simulink model "model_try"  (R2025b)
settings: Solver=VariableStepAuto  StartTime=0.0  StopTime=5.0  RelTol=1e-3
undefined symbols (not defined in the file or in its folder): g, pow, R0
settings Model: SimulationMode=rapid-accelerator  Creator=velo  LastModifiedBy=velo

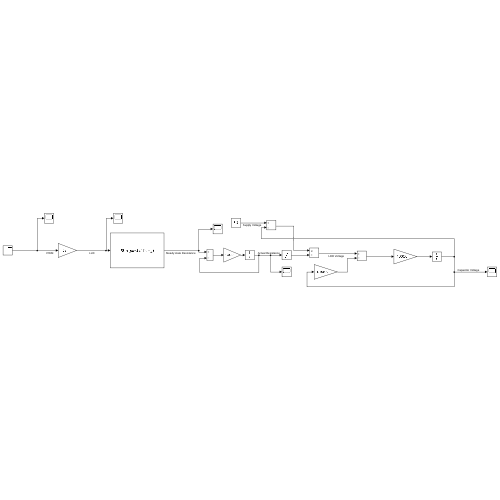
[thumbnail: Simulink's stored preview of the top-level diagram]
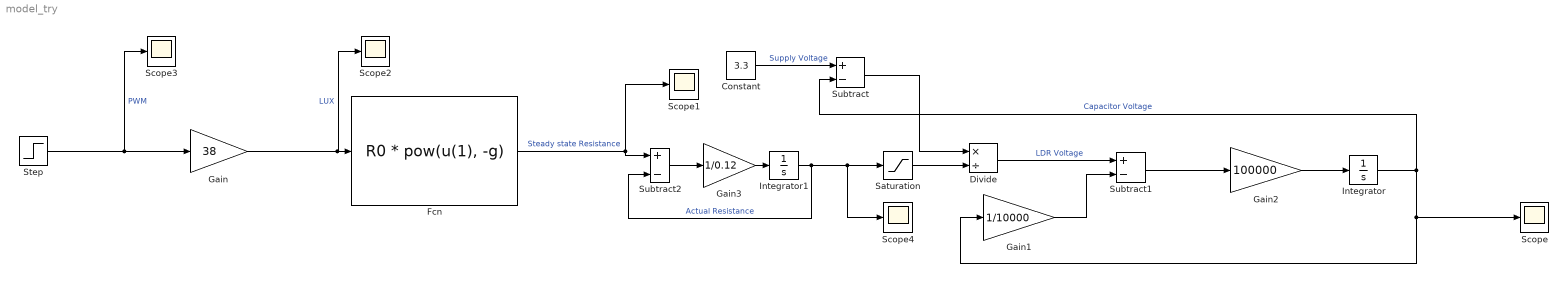
== system model_try ==
  Constant : Constant  Value=3.3
  Divide : Product  Inputs=*/
  Fcn : Fcn  Expr=R0 * pow(u(1), -g)
  Gain : Gain  Gain=38
  Gain1 : Gain  Gain=1/10000
  Gain2 : Gain  Gain=100000
  Gain3 : Gain  Gain=1/0.12
  Integrator : Integrator  InitialCondition=0.255
  Integrator1 : Integrator  InitialCondition=120000
  Saturation : Saturate  UpperLimit=inf  LowerLimit=100
  Scope{,1..4} (5 alike) : Scope
      Scope settings: ActiveDisplayYMinimum=0.22586838074123314  ActiveDisplayYMaximum=0.44234428417345445
      Scope1 settings: ActiveDisplayYMinimum=62371.168073078486  ActiveDisplayYMaximum=126049.34258955714
      Scope2 settings: ActiveDisplayYMinimum=16.625  ActiveDisplayYMaximum=40.375  DataLoggingVariableName=ScopeData2
      Scope3 settings: ActiveDisplayYMinimum=-1  ActiveDisplayYMaximum=1  DataLoggingVariableName=ScopeData3
      Scope4 settings: ActiveDisplayYMinimum=62331.451558114684  ActiveDisplayYMaximum=126407.61649354281  DataLoggingVariableName=ScopeData4
  Step : Step  Before=0.5  SampleTime=1
  Subtract : Sum  Inputs=+-
  Subtract1 : Sum  Inputs=+-
  Subtract2 : Sum  Inputs=+-
  wires:
  Step/1 -> Gain/1, Scope3/1  "PWM"
  Gain/1 -> Scope2/1, Fcn/1  "LUX"
  Constant/1 -> Subtract/1  "Supply Voltage"
  Subtract/1 -> Divide/1
  Divide/1 -> Subtract1/1  "LDR Voltage"
  Gain1/1 -> Subtract1/2
  Subtract1/1 -> Gain2/1
  Gain2/1 -> Integrator/1
  Integrator/1 -> Subtract/2, Scope/1, Gain1/1  "Capacitor Voltage"
  Fcn/1 -> Subtract2/1, Scope1/1  "Steady state Resistance"
  Saturation/1 -> Divide/2
  Subtract2/1 -> Gain3/1
  Gain3/1 -> Integrator1/1
  Integrator1/1 -> Subtract2/2, Scope4/1, Saturation/1  "Actual Resistance"
